simulink model "eml_2nd_order_filter_vectorized"  (Simulink 7.7)
settings: Solver=FixedStepDiscrete  StartTime=0.0  StopTime=0  RelTol=1e-3
values from neighbouring files (symbols this model uses):
  den = [1                  -1.4542435862515900  0.5740619150839550]    [fi_instrumentation_fixed_point_filter_demo.m]
  num = [0.0299545822080925  0.0599091644161849  0.0299545822080925]    [fi_instrumentation_fixed_point_filter_demo.m]
settings Model: Creator=tbryan  LastModifiedBy=kbackhou  ExtModeAutoUpdateStatusClock=off
settings OptimizationCC: InitFltsAndDblsToZero=on
settings DebuggingCC: ArtificialAlgebraicLoopMsg=none  SignalResolutionControl=TryResolveAllWithWarning  SolverPrmCheckMsg=none  InheritedTsInSrcMsg=none  DiscreteInheritContinuousMsg=none  MultiTaskDSMMsg=warning  MultiTaskCondExecSysMsg=none  MultiTaskRateTransMsg=warning  TasksWithSamePriorityMsg=none  SigSpecEnsureSampleTimeMsg=none  IntegerOverflowMsg=none  Int32ToFloatConvMsg=none  ParameterDowncastMsg=none  ParameterOverflowMsg=none  ParameterPrecisionLossMsg=none  UnknownTsInhSupMsg=none  StrictBusMsg=Warning
settings SFSimCC: SFSimOverflowDetection=off  SimParseCustomCode=off
settings RTWCC: GenerateReport=on  LaunchReport=on  IncludeERTFirstTime=on

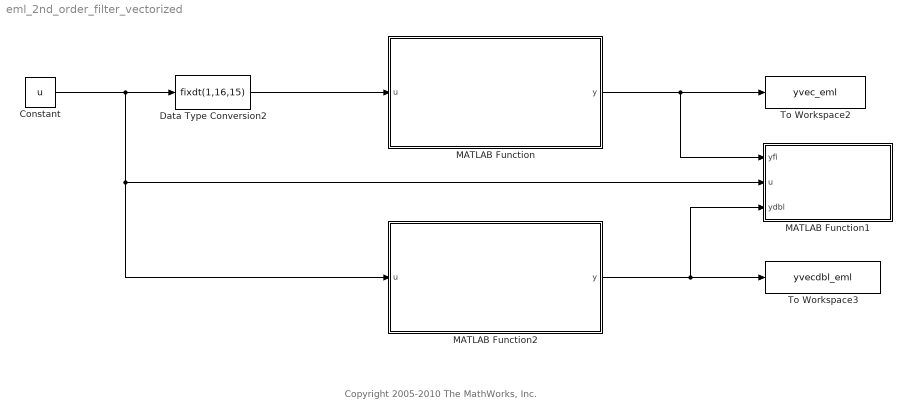
== system eml_2nd_order_filter_vectorized ==
  note: Copyright 2005-2010 The MathWorks, Inc.
  Constant : Constant  Value=u  OutDataTypeStr=double
  Data Type Conversion2 : DataTypeConversion  OutDataTypeStr=fixdt(1,16,15)  RndMeth=Nearest  SaturateOnIntegerOverflow=on
  MATLAB Function : Stateflow chart  TreatAsAtomicUnit=on
  MATLAB Function1 : Stateflow chart  TreatAsAtomicUnit=on
  MATLAB Function2 : Stateflow chart  TreatAsAtomicUnit=on
  To Workspace2 : ToWorkspace  VariableName=yvec_eml  SampleTime=-1  SaveFormat=Array
      settings: MaxDataPoints=1
  To Workspace3 : ToWorkspace  VariableName=yvecdbl_eml  SampleTime=-1  SaveFormat=Array
      settings: MaxDataPoints=1
  wires:
  Constant/1 -> Data Type Conversion2/1, MATLAB Function1/2(u), MATLAB Function2/1(u)
  Data Type Conversion2/1 -> MATLAB Function/1(u)
  MATLAB Function/1(y) -> To Workspace2/1, MATLAB Function1/1(yfi)
  MATLAB Function2/1(y) -> To Workspace3/1, MATLAB Function1/3(ydbl)

== matlab function MATLAB Function1 ==
  settings: fimath=|
      | fimath('RoundMode',             'floor', ...
      |            'OverflowMode',          'wrap', ...
      |            'ProductMode',           'SpecifyPrecision', ...
      |            'ProductWordLength',     32, ...
      |            'ProductFractionLength', 30, ...
      |            'SumMode',               'SpecifyPrecision', ...
      |            'SumWordLength',         32, ...
      |            'SumFractionLength',     30)
  data: yfi input double; u input double; ydbl input double; num parameter double; den parameter double
function vector_plot(yfi, u, ydbl, num, den)
%#codegen

eml.extrinsic('fi_datatype_override_demo_plot');

fi_datatype_override_demo_plot(num,den,u,yfi,ydbl,'MATLAB Function Block Case')

== matlab function MATLAB Function2 ==
  settings: fimath=fimath;
  data: num parameter double; den parameter double; u input double; y output double
function y = fi_2nd_order_filter(num, den, u)
%#codegen

y = fieml_2nd_order_filter(num,den,u);

== matlab function MATLAB Function ==
  settings: fimath=fimath;
  data: num parameter double; den parameter double; u input double; y output double
function y = fi_2nd_order_filter(num, den, u)
%#codegen

y = fieml_2nd_order_filter(num,den,u);
